simulink model "AC_SYS_SS"  (R2023b)
settings: Solver=FixedStepDiscrete  StartTime=0.0  StopTime=2  FixedStep=Ts_Power  RelTol=1e-4  EnableMultiTasking=on
PreLoadFcn:
  | HVDCMMCInterconnectionParam
StartFcn:
  | tic
StopFcn:
  | toc
values from neighbouring files (symbols this model uses):
  C_PM = 1.758e-3    (= 0.001758)    [HVDCMMCInterconnectionParam.m]
  D_R = 0.001    [HVDCMMCInterconnectionParam.m]
  D_Rs = 1e8    (= 100000000)    [HVDCMMCInterconnectionParam.m]
  Fnom = 50    [HVDCMMCInterconnectionParam.m]
  HRM = 2    [HVDCMMCInterconnectionParam.m]
  Limits_Qreg = [ 0.25, -0.25 ]    [HVDCMMCInterconnectionParam.m]
  Nb_PM = 36    [HVDCMMCInterconnectionParam.m]
  P_Ld1 = Psc/30    (= 666666666.667)    [HVDCMMCInterconnectionParam.m]
  Slope_Pref = 0.5    [HVDCMMCInterconnectionParam.m]
  Slope_Qref = 0.5    [HVDCMMCInterconnectionParam.m]
  Slope_Vdc_ref = Vnom_dc/5    (= 128000)    [HVDCMMCInterconnectionParam.m]
  Tbrk1_On = 0.1    [HVDCMMCInterconnectionParam.m]
  Tbrk2_On = 1.0    (= 1)    [HVDCMMCInterconnectionParam.m]
  Tdeblock = 1.5    [HVDCMMCInterconnectionParam.m]
  Tfault = 9999    [HVDCMMCInterconnectionParam.m]
  Ton_Converter2 = 4    [HVDCMMCInterconnectionParam.m]
  Ton_PQreg = 4    [HVDCMMCInterconnectionParam.m]
  Ton_VDCreg = 1.5    [HVDCMMCInterconnectionParam.m]
  Ts = Ts_Control    (= 4e-05)    [HVDCMMCInterconnectionParam.m]
  Ts_Power = 20e-6    (= 2e-05)    [HVDCMMCInterconnectionParam.m]
  Vb_dc = Vnom_dc    (= 640000)    [HVDCMMCInterconnectionParam.m]
  Vnom_dc = 640e3    (= 640000)    [HVDCMMCInterconnectionParam.m]
  Vnom_prim = 400e3    (= 400000)    [HVDCMMCInterconnectionParam.m]
  Vnom_sec = 333e3    (= 333000)    [HVDCMMCInterconnectionParam.m]
  w = 2*pi*Fnom    (= 314.159265359)    [HVDCMMCInterconnectionParam.m]
undefined symbols (not defined in the file or in its folder): ACSYS_T, DiscIntNeverNeededParam, Discrete, Pcc, sps_AC, spsDiodeModel
libraries: simulink x12, spsThreePhaseSeriesRLCBranchLib x7, spsGroundLib x3, spsControlledVoltageSourceLib x3, spsMultimeterLib x2, spsThreePhaseVIMeasurementLib x2, spsThreePhaseBreakerLib x1, spsThreePhaseSeriesRLCLoadLib x1, spspowerguiLib x1
(part 2 of 2)

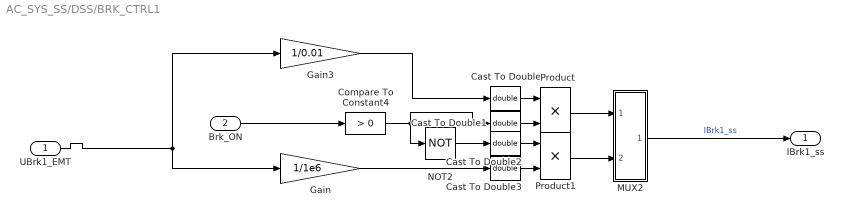
== system AC_SYS_SS/DSS/BRK_CTRL1 ==
  UBrk1_EMT : Inport
  Brk_ON : Inport  Port=2
  Cast To Double{,1..3} (4 alike) : DataTypeConversion  OutDataTypeStr=double  SaturateOnIntegerOverflow=off  RndMeth=Floor
  Compare To Constant4 : simulink/Logic and Bit Operations/Compare To Constant  relop=>  const=0  OutDataTypeStr=boolean
  Gain : Gain  Gain=1/1e6
  Gain3 : Gain  Gain=1/0.01
  MUX2 : Subsystem
  NOT2 : Logic  Operator=NOT  IconShape=distinctive  AllPortsSameDT=off  OutDataTypeStr=boolean
  Product : Product
  Product1 : Product
  IBrk1_ss : Outport
  wires:
  Cast To Double1/1 -> Product/2
  Product1/1 -> MUX2/2(In2)
  UBrk1_EMT/1 -> Gain3/1, Gain/1
  Compare To Constant4/1 -> Cast To Double1/1, NOT2/1
  Product/1 -> MUX2/1(In1)
  Gain/1 -> Cast To Double3/1
  NOT2/1 -> Cast To Double2/1
  Cast To Double/1 -> Product/1
  Gain3/1 -> Cast To Double/1
  Cast To Double3/1 -> Product1/2
  Brk_ON/1 -> Compare To Constant4/1
  Cast To Double2/1 -> Product1/1
  MUX2/1(Out1) -> IBrk1_ss/1  "IBrk1_ss"

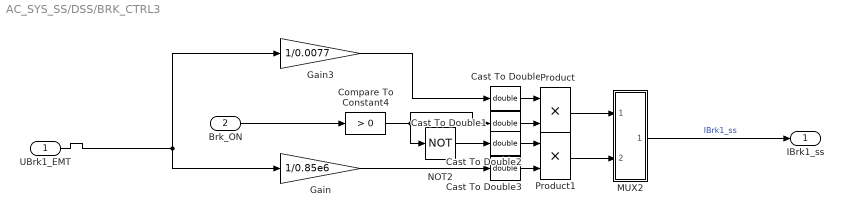
== system AC_SYS_SS/DSS/BRK_CTRL3 ==
  UBrk1_EMT : Inport
  Brk_ON : Inport  Port=2
  Cast To Double{,1..3} (4 alike) : DataTypeConversion  OutDataTypeStr=double  SaturateOnIntegerOverflow=off  RndMeth=Floor
  Compare To Constant4 : simulink/Logic and Bit Operations/Compare To Constant  relop=>  const=0  OutDataTypeStr=boolean
  Gain : Gain  Gain=1/0.85e6
  Gain3 : Gain  Gain=1/0.0077
  MUX2 : Subsystem
  NOT2 : Logic  Operator=NOT  IconShape=distinctive  AllPortsSameDT=off  OutDataTypeStr=boolean
  Product : Product
  Product1 : Product
  IBrk1_ss : Outport
  wires:
  Cast To Double1/1 -> Product/2
  Product1/1 -> MUX2/2(In2)
  UBrk1_EMT/1 -> Gain3/1, Gain/1
  Compare To Constant4/1 -> Cast To Double1/1, NOT2/1
  Product/1 -> MUX2/1(In1)
  Gain/1 -> Cast To Double3/1
  NOT2/1 -> Cast To Double2/1
  Cast To Double/1 -> Product/1
  Gain3/1 -> Cast To Double/1
  Cast To Double3/1 -> Product1/2
  Brk_ON/1 -> Compare To Constant4/1
  Cast To Double2/1 -> Product1/1
  MUX2/1(Out1) -> IBrk1_ss/1  "IBrk1_ss"

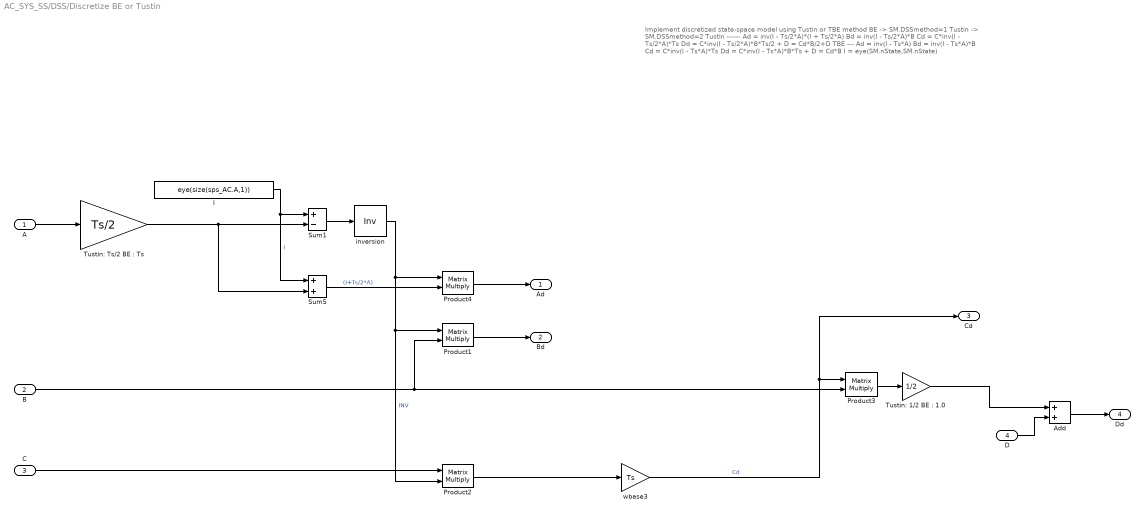
== system AC_SYS_SS/DSS/Discretize BE or Tustin ==
  note: Implement discretized state-space model using Tustin or TBE method
      |
      | BE      -> SM.DSSmethod=1
      | Tustin  -> SM.DSSmethod=2
      |
      |
      | Tustin
      | ------
      | Ad = inv(I - Ts/2*A)*(I + Ts/2*A)
      | Bd = inv(I - Ts/2*A)*B
      | Cd = C*inv(I - Ts/2*A)*Ts
      | Dd = C*inv(I - Ts/2*A)*B*Ts/2  + D  =  Cd*B/2+D
      |
      | TBE
      | ---
      | Ad = inv(I - Ts*A)
      | Bd = inv(I - Ts*A)*B
      | Cd = C*inv(I - Ts*A)*Ts
      | Dd = C*inv(I - Ts*A)*B*Ts  + D  =  Cd*B
      |
      | I = eye(SM.nState,SM.nState)
  A : Inport
  B : Inport  Port=2
  C : Inport  Port=3
  D : Inport  Port=4
  Add : Sum
  I : Constant  Value=eye(size(sps_AC.A,1))
  Product{1..4} (4 alike) : Product  Multiplication=Matrix(*)  SaturateOnIntegerOverflow=on  OutDataTypeStr=Inherit: Same as first input
  Sum1 : Sum  Inputs=+-  SaturateOnIntegerOverflow=on
  Sum5 : Sum  SaturateOnIntegerOverflow=on
  "Tustin: 1/2 BE : 1.0" : Gain  Gain=1/2  SaturateOnIntegerOverflow=on  OutDataTypeStr=Inherit: Same as input  ParamDataTypeStr=Inherit: Same as input
  "Tustin: Ts/2 BE : Ts" : Gain  Gain=Ts/2  SaturateOnIntegerOverflow=on  OutDataTypeStr=Inherit: Same as input  ParamDataTypeStr=Inherit: Same as input
  inversion : Product  Inputs=/  Multiplication=Matrix(*)  RndMeth=Zero
  wbase3 : Gain  Gain=Ts  SaturateOnIntegerOverflow=on  OutDataTypeStr=Inherit: Same as input  ParamDataTypeStr=Inherit: Same as input
  Ad : Outport  VectorParamsAs1DForOutWhenUnconnected=off
  Bd : Outport  Port=2  VectorParamsAs1DForOutWhenUnconnected=off
  Cd : Outport  Port=3  VectorParamsAs1DForOutWhenUnconnected=off
  Dd : Outport  Port=4  VectorParamsAs1DForOutWhenUnconnected=off
  wires:
  wbase3/1 -> Product3/1, Cd/1  "Cd"
  Product2/1 -> wbase3/1
  "Tustin: 1/2 BE : 1.0"/1 -> Add/1
  Product3/1 -> "Tustin: 1/2 BE : 1.0"/1
  C/1 -> Product2/1
  B/1 -> Product3/2, Product1/2
  Product1/1 -> Bd/1
  Sum5/1 -> Product4/2  "(I+Ts/2*A)"
  inversion/1 -> Product4/1, Product1/1, Product2/2  "INV"
  Sum1/1 -> inversion/1
  I/1 -> Sum1/1, Sum5/1  "I"
  A/1 -> "Tustin: Ts/2 BE : Ts"/1
  Product4/1 -> Ad/1
  "Tustin: Ts/2 BE : Ts"/1 -> Sum5/2, Sum1/2
  Add/1 -> Dd/1
  D/1 -> Add/2

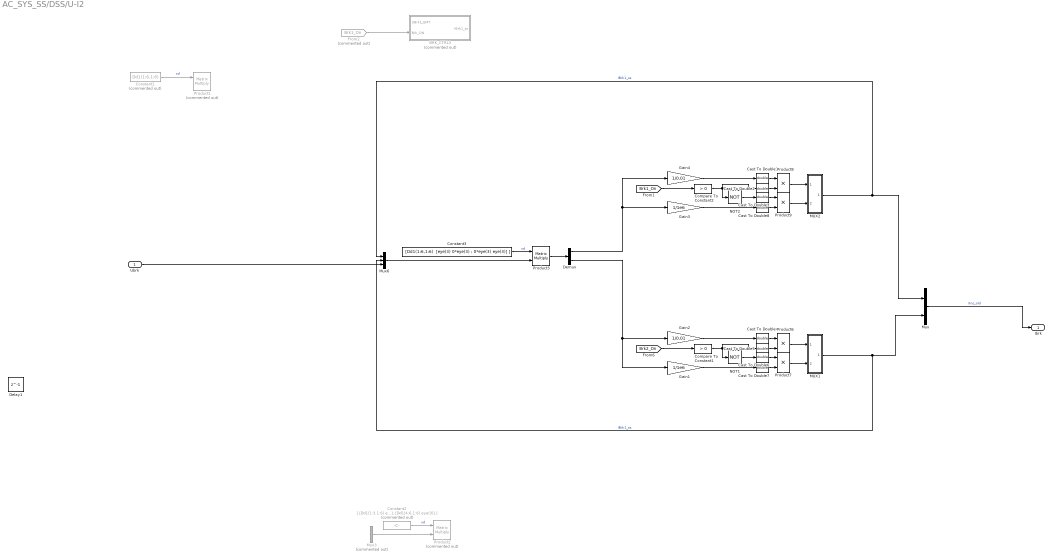
== system AC_SYS_SS/DSS/U-I2 ==
  Ubrk : Inport
  BRK_CTRL3 : Subsystem  Commented=on
  Cast To Double{1..8} (8 alike) : DataTypeConversion  OutDataTypeStr=double  SaturateOnIntegerOverflow=off  RndMeth=Floor
  Compare To Constant1 : simulink/Logic and Bit Operations/Compare To Constant  relop=>  const=0  OutDataTypeStr=boolean
  Compare To Constant2 : simulink/Logic and Bit Operations/Compare To Constant  relop=>  const=0  OutDataTypeStr=boolean
  Constant1 : Constant  Commented=on  Value=Dd1(1:6,1:6)
  Constant2 : Constant  Commented=on  Value=[ [Dd1(1:3,1:6) eye(3)]; [Dd1(4:6,1:6) eye(3)] ]
  Constant3 : Constant  Value="[Dd1(1:6,1:6)  [eye(3) 0*eye(3) ; 0*eye(3) eye(3)] ]"
  Delay1 : Delay  DelayLength=1  SampleTime=Ts_Power
  Demux : Demux  Outputs=2
  From2 : From  Commented=on  GotoTag=Brk1_On  TagVisibility=global
  Gain1 : Gain  Gain=1/1e6
  Gain2 : Gain  Gain=1/0.01
  Gain3 : Gain  Gain=1/1e6
  Gain4 : Gain  Gain=1/0.01
  MUX1 : Subsystem
  MUX2 : Subsystem
  Mux : Mux  Inputs=2
  Mux3 : Mux  Commented=on  Inputs=2
  Mux6 : Mux  Inputs=3
  NOT1 : Logic  Operator=NOT  IconShape=distinctive  AllPortsSameDT=off  OutDataTypeStr=boolean
  NOT2 : Logic  Operator=NOT  IconShape=distinctive  AllPortsSameDT=off  OutDataTypeStr=boolean
  Product1 : Product  Commented=on  Multiplication=Matrix(*)  SaturateOnIntegerOverflow=on  OutDataTypeStr=Inherit: Same as first input
  Product2 : Product  Commented=on  Multiplication=Matrix(*)  SaturateOnIntegerOverflow=on  OutDataTypeStr=Inherit: Same as first input
  Product3 : Product  Multiplication=Matrix(*)  SaturateOnIntegerOverflow=on  OutDataTypeStr=Inherit: Same as first input
  Product{6..9} (4 alike) : Product
  Ibrk : Outport
  wires:
  Mux/1 -> Ibrk/1  "Xns_old"
  Constant1/1 -> Product1/1  "xd"
  Cast To Double7/1 -> Product7/2
  Cast To Double6/1 -> Product7/1
  Gain2/1 -> Cast To Double4/1
  Compare To Constant1/1 -> Cast To Double5/1, NOT1/1
  NOT1/1 -> Cast To Double6/1
  Gain1/1 -> Cast To Double7/1
  Cast To Double5/1 -> Product6/2
  Cast To Double4/1 -> Product6/1
  [Brk2_On] -> Compare To Constant1/1
  Demux/2 -> Gain1/1, Gain2/1
  MUX1/1(UBrk1_EMT) -> Mux6/2, Mux/2  "IBrk1_ss"
  Product6/1 -> MUX1/1(In1)
  Product7/1 -> MUX1/2(In2)
  From2/1 -> BRK_CTRL3/2(Brk_ON)
  Cast To Double1/1 -> Product8/1
  Cast To Double2/1 -> Product8/2
  Gain3/1 -> Cast To Double8/1
  NOT2/1 -> Cast To Double3/1
  Cast To Double8/1 -> Product9/2
  Cast To Double3/1 -> Product9/1
  [Brk1_On] -> Compare To Constant2/1
  MUX2/1(UBrk1_EMT) -> Mux6/1, Mux/1  "IBrk1_ss"
  Gain4/1 -> Cast To Double1/1
  Product8/1 -> MUX2/1(In1)
  Compare To Constant2/1 -> Cast To Double2/1, NOT2/1
  Product9/1 -> MUX2/2(In2)
  ? -> Mux3/1
  ? -> Mux3/2
  Mux3/1 -> Product2/2
  Constant2/1 -> Product2/1  "xd"
  Mux6/1 -> Product3/2
  Constant3/1 -> Product3/1  "xd"
  Product3/1 -> Demux/1
  Demux/1 -> Gain4/1, Gain3/1
  Ubrk/1 -> Mux6/3

== system AC_SYS_SS/DSS/BRK_CTRL1/MUX2 ==
  In1 : Inport
  In2 : Inport  Port=2
  Demux4 : Demux  Outputs=3
  Demux5 : Demux  Outputs=3
  Mux13 : Mux  Inputs=2
  Mux14 : Mux  Inputs=2
  Mux15 : Mux  Inputs=3
  Mux8 : Mux  Inputs=2
  Sum1 : Sum  Inputs=1  InputSameDT=on  SaturateOnIntegerOverflow=on  OutDataTypeStr=Inherit: Same as first input
  Sum4 : Sum  Inputs=1  InputSameDT=on  SaturateOnIntegerOverflow=on  OutDataTypeStr=Inherit: Same as first input
  Sum5 : Sum  Inputs=1  InputSameDT=on  SaturateOnIntegerOverflow=on  OutDataTypeStr=Inherit: Same as first input
  Out1 : Outport
  wires:
  Demux5/3 -> Mux14/2
  In1/1 -> Demux4/1
  Demux4/1 -> Mux8/1
  Demux5/1 -> Mux8/2
  In2/1 -> Demux5/1
  Sum1/1 -> Mux15/1
  Demux5/2 -> Mux13/2
  Mux14/1 -> Sum5/1
  Mux8/1 -> Sum1/1
  Demux4/2 -> Mux13/1
  Mux13/1 -> Sum4/1
  Sum5/1 -> Mux15/3
  Sum4/1 -> Mux15/2
  Demux4/3 -> Mux14/1
  Mux15/1 -> Out1/1

== system AC_SYS_SS/DSS/BRK_CTRL3/MUX2 ==
  In1 : Inport
  In2 : Inport  Port=2
  Demux4 : Demux  Outputs=3
  Demux5 : Demux  Outputs=3
  Mux13 : Mux  Inputs=2
  Mux14 : Mux  Inputs=2
  Mux15 : Mux  Inputs=3
  Mux8 : Mux  Inputs=2
  Sum1 : Sum  Inputs=1  InputSameDT=on  SaturateOnIntegerOverflow=on  OutDataTypeStr=Inherit: Same as first input
  Sum4 : Sum  Inputs=1  InputSameDT=on  SaturateOnIntegerOverflow=on  OutDataTypeStr=Inherit: Same as first input
  Sum5 : Sum  Inputs=1  InputSameDT=on  SaturateOnIntegerOverflow=on  OutDataTypeStr=Inherit: Same as first input
  Out1 : Outport
  wires:
  Demux5/3 -> Mux14/2
  In1/1 -> Demux4/1
  Demux4/1 -> Mux8/1
  Demux5/1 -> Mux8/2
  In2/1 -> Demux5/1
  Sum1/1 -> Mux15/1
  Demux5/2 -> Mux13/2
  Mux14/1 -> Sum5/1
  Mux8/1 -> Sum1/1
  Demux4/2 -> Mux13/1
  Mux13/1 -> Sum4/1
  Sum5/1 -> Mux15/3
  Sum4/1 -> Mux15/2
  Demux4/3 -> Mux14/1
  Mux15/1 -> Out1/1

== system AC_SYS_SS/DSS/U-I2/BRK_CTRL3 ==
  UBrk1_EMT : Inport
  Brk_ON : Inport  Port=2
  Cast To Double{,1..3} (4 alike) : DataTypeConversion  OutDataTypeStr=double  SaturateOnIntegerOverflow=off  RndMeth=Floor
  Compare To Constant4 : simulink/Logic and Bit Operations/Compare To Constant  relop=>  const=0  OutDataTypeStr=boolean
  Gain : Gain  Gain=1/1e6
  Gain3 : Gain  Gain=1/0.01
  MUX2 : Subsystem
  NOT2 : Logic  Operator=NOT  IconShape=distinctive  AllPortsSameDT=off  OutDataTypeStr=boolean
  Product : Product
  Product1 : Product
  IBrk1_ss : Outport
  wires:
  Cast To Double1/1 -> Product/2
  Product1/1 -> MUX2/2(In2)
  UBrk1_EMT/1 -> Gain3/1, Gain/1
  Compare To Constant4/1 -> Cast To Double1/1, NOT2/1
  Product/1 -> MUX2/1(In1)
  Gain/1 -> Cast To Double3/1
  NOT2/1 -> Cast To Double2/1
  Cast To Double/1 -> Product/1
  Gain3/1 -> Cast To Double/1
  Cast To Double3/1 -> Product1/2
  Brk_ON/1 -> Compare To Constant4/1
  Cast To Double2/1 -> Product1/1
  MUX2/1(Out1) -> IBrk1_ss/1  "IBrk1_ss"

== system AC_SYS_SS/DSS/U-I2/MUX1 ==
  In1 : Inport
  In2 : Inport  Port=2
  Demux4 : Demux  Outputs=3
  Demux5 : Demux  Outputs=3
  Mux13 : Mux  Inputs=2
  Mux14 : Mux  Inputs=2
  Mux15 : Mux  Inputs=3
  Mux8 : Mux  Inputs=2
  Sum1 : Sum  Inputs=1  InputSameDT=on  SaturateOnIntegerOverflow=on  OutDataTypeStr=Inherit: Same as first input
  Sum4 : Sum  Inputs=1  InputSameDT=on  SaturateOnIntegerOverflow=on  OutDataTypeStr=Inherit: Same as first input
  Sum5 : Sum  Inputs=1  InputSameDT=on  SaturateOnIntegerOverflow=on  OutDataTypeStr=Inherit: Same as first input
  UBrk1_EMT : Outport
  wires:
  Demux5/3 -> Mux14/2
  In1/1 -> Demux4/1
  Demux4/1 -> Mux8/1
  Demux5/1 -> Mux8/2
  In2/1 -> Demux5/1
  Sum1/1 -> Mux15/1
  Demux5/2 -> Mux13/2
  Mux14/1 -> Sum5/1
  Mux8/1 -> Sum1/1
  Demux4/2 -> Mux13/1
  Mux13/1 -> Sum4/1
  Sum5/1 -> Mux15/3
  Sum4/1 -> Mux15/2
  Demux4/3 -> Mux14/1
  Mux15/1 -> UBrk1_EMT/1

== system AC_SYS_SS/DSS/U-I2/MUX2 ==
  In1 : Inport
  In2 : Inport  Port=2
  Demux4 : Demux  Outputs=3
  Demux5 : Demux  Outputs=3
  Mux13 : Mux  Inputs=2
  Mux14 : Mux  Inputs=2
  Mux15 : Mux  Inputs=3
  Mux8 : Mux  Inputs=2
  Sum1 : Sum  Inputs=1  InputSameDT=on  SaturateOnIntegerOverflow=on  OutDataTypeStr=Inherit: Same as first input
  Sum4 : Sum  Inputs=1  InputSameDT=on  SaturateOnIntegerOverflow=on  OutDataTypeStr=Inherit: Same as first input
  Sum5 : Sum  Inputs=1  InputSameDT=on  SaturateOnIntegerOverflow=on  OutDataTypeStr=Inherit: Same as first input
  UBrk1_EMT : Outport
  wires:
  Demux5/3 -> Mux14/2
  In1/1 -> Demux4/1
  Demux4/1 -> Mux8/1
  Demux5/1 -> Mux8/2
  In2/1 -> Demux5/1
  Sum1/1 -> Mux15/1
  Demux5/2 -> Mux13/2
  Mux14/1 -> Sum5/1
  Mux8/1 -> Sum1/1
  Demux4/2 -> Mux13/1
  Mux13/1 -> Sum4/1
  Sum5/1 -> Mux15/3
  Sum4/1 -> Mux15/2
  Demux4/3 -> Mux14/1
  Mux15/1 -> UBrk1_EMT/1

== system AC_SYS_SS/DSS/U-I2/BRK_CTRL3/MUX2 ==
  In1 : Inport
  In2 : Inport  Port=2
  Demux4 : Demux  Outputs=3
  Demux5 : Demux  Outputs=3
  Mux13 : Mux  Inputs=2
  Mux14 : Mux  Inputs=2
  Mux15 : Mux  Inputs=3
  Mux8 : Mux  Inputs=2
  Sum1 : Sum  Inputs=1  InputSameDT=on  SaturateOnIntegerOverflow=on  OutDataTypeStr=Inherit: Same as first input
  Sum4 : Sum  Inputs=1  InputSameDT=on  SaturateOnIntegerOverflow=on  OutDataTypeStr=Inherit: Same as first input
  Sum5 : Sum  Inputs=1  InputSameDT=on  SaturateOnIntegerOverflow=on  OutDataTypeStr=Inherit: Same as first input
  Out1 : Outport
  wires:
  Demux5/3 -> Mux14/2
  In1/1 -> Demux4/1
  Demux4/1 -> Mux8/1
  Demux5/1 -> Mux8/2
  In2/1 -> Demux5/1
  Sum1/1 -> Mux15/1
  Demux5/2 -> Mux13/2
  Mux14/1 -> Sum5/1
  Mux8/1 -> Sum1/1
  Demux4/2 -> Mux13/1
  Mux13/1 -> Sum4/1
  Sum5/1 -> Mux15/3
  Sum4/1 -> Mux15/2
  Demux4/3 -> Mux14/1
  Mux15/1 -> Out1/1

== matlab function AC_SYS_SS/MATLAB Function ==
  data: usw output; Id input; status output; Vd input
function [usw, status]   = DFcn(Id, Vd)

    persistent SW;
    
    if(isempty(SW)) SW = 1; end
    
    
    if(Id<=0 && SW == 1)
    
        SW = 0;
    elseif( (Id>0 && SW == 0) || (Vd > 0.7 && SW == 0 && Id>eps) )
        SW = 1;
    end
    
    status = SW;
    usw = Vd;

end

== matlab function AC_SYS_SS/MATLAB Function2 ==
  data: Usm input; Uref input; UDt output; Stt output; Ip input; Ic input; UDb output; Stb output; IDt output; IDb output; Vbl output; Ts parameter; D_R parameter; D_Rs parameter; Nb_SM parameter; C parameter; Vin output
function [UDt, Stt, UDb, Stb, IDt, IDb, Vbl, Vin]   = DFcn(Usm, Uref, Ip, Ic, Ts, D_R, D_Rs, Nb_SM, C)

    UDt = 0; UDb = 0; Stt = 0; Stb = 0;

    Ib    = 0;
    Vbl = 0;
    Vin = 0;
    IDt = 0;
    IDb = 0;
    
    persistent timer;
    persistent Usm_old;
    persistent Ip_old;
    persistent Ic_old;
    persistent SWt;
    persistent SWb;

    persistent Uc_old;
    persistent Uc;
    persistent x_old;
    persistent Req;
    
    if(isempty(timer)) 
        timer = 0; 
        Usm_old = 0;
        Ip_old = 0;
        Ic_old = 0;
        SWt = 0;
        SWb = 0;
        Uc_old = 0;
        Uc = 0;
        x_old = 0;
        Req = D_R*D_Rs/(D_R+D_Rs);
    end
    
    timer = timer + Ts;

%%%%%%%%%%%%%%% Calc Vin & Vbl %%%%%%%%%%%%%%%
    %x = Nb_SM*(Ip_old*Uref(1)+Ic_old*Uref(2))/(C*Nb_SM);
    x = Nb_SM*(Ip*Uref(1)+Ic*Uref(2))/(C*Nb_SM);

    Uc = (Ts/2)*(x+x_old) + Uc_old;
    
    Vin = Uc*Uref(1)*Nb_SM;
    Vbl = Uc*Uref(2)*Nb_SM;


    x_old = x;
    Uc_old = Uc;
%%%%%%%%%%%%%%%%%%%%%%%%%%%%%%


    Ib = Ip-D_Rs/(D_R+D_Rs)*Ic;


    if(Uref(2) > 0)

        if(Ic < 0)
            UDt = Usm - Vbl;
        else
            UDt = Ic*Req;
        end
    
        if(Ib > 0)
            UDb = -Usm;
        else
            UDb = -Ib*Req;
        end

        1==1;
    
        if(-0.0001 + D_Rs/(D_R+D_Rs)*Ic_old <= 0 && SWt == 1)
            SWt = 0;
        elseif(-0.0001 + D_Rs/(D_R+D_Rs)*Ic > 0 && SWt == 0) 
            SWt = 1;
        end
    
        if(Ib<=0 && SWb == 0 && SWt == 0)
            SWb = 1;
        elseif( (Ib > -eps && SWb == 1 && Vbl > 0 && Ip < 0))
            SWb = 0;
        end

    else
        UDt =  Ip*(D_Rs/2)*D_R/(D_Rs/2+D_R);
        UDb = -UDt;


        if((0.1+Ib<=0 || Ip<0) && SWb == 0)
            SWb = 1;
            SWt = 0;
        elseif( (Ip>0 || -0.1 + Ic >= 0) && SWb == 1)
            SWb = 0;
            SWt = 1;
        end


    end




    IDt = SWt * UDt / D_R;
    if(IDt<0) IDt = 0; end

    IDb = SWb * UDb / D_R;
    if(IDb<0) IDb = 0; end


    Usm_old = Usm;
    Ip_old = Ip;
    Ic_old = Ic;



    Stt =  SWt;
    Stb = SWb;

end


    % if(SWt>0.5)
    %     IDt = UDt / D_R;
    %     if(IDt<0) IDt = 0; end
    % else
    %     IDt = 0;
    % end
    % 
    % if(SWb>0.5)
    %     IDb = UDb / D_R;
    %     if(IDb<0) IDb = 0; end
    % else
    %     IDb = 0;
    % end


    % persistent SW;
    % 
    % if(isempty(SW)) SW = 1; end
    % 
    % 
    % if(Id<=0 && SW == 1)
    % 
    %     SW = 0;
    % elseif( (Id>0 && SW == 0) || (Vd > 0 && SW == 0 && Id>eps) )
    %     SW = 1;
    % end
    % 
    % status = SW;
    % usw = Vd;

== matlab function AC_SYS_SS/DQn->ABC ==
  settings: updateMethod=DISCRETE
  data: Xdcpnz_c input; tho input; Xabc output; N parameter
%function abc = Mult(Z0,Zdp,Zqp,Zdn,Zqn,Zdz,Zqz,th, N)
function Xabc = dqn2abc(Xdcpnz_c,tho,N)

    persistent Sas;
    persistent Ssa;

    if(isempty(Sas)) 
        a = -0.5+0.866i;
        a2 = -0.5-0.866i;
        Sas = [1,a,a2;1,a2,a;1,1,1]/3;
        Ssa = eye(3)/(Sas);
    end

    Xabc = zeros(3,1);

    for i = 1 : N+1
    
    
        if(i>1)
            h = i-1;
    
            th = h*tho;
        
            mag_p = abs(Xdcpnz_c(1,i));
            ang_p = angle(Xdcpnz_c(1,i));
            mag_n = abs(Xdcpnz_c(2,i));
            ang_n = angle(Xdcpnz_c(2,i));
            mag_z = abs(Xdcpnz_c(3,i));
            ang_z = angle(Xdcpnz_c(3,i));
            
            abc3p = mag_p*[sin(th+ang_p) ; sin(th+ang_p-2*pi/3) ; sin(th+ang_p+2*pi/3) ];
            abc3n = mag_n*[sin(th+ang_n) ; sin(th+ang_n+2*pi/3) ; sin(th+ang_n-2*pi/3) ];
            abc3z = mag_z*[sin(th+ang_z) ; sin(th+ang_z)        ; sin(th+ang_z)  ];
        
            Xabc = Xabc + abc3p+abc3n+abc3z;
        else
            Xabc = Xabc + real(Ssa*(Xdcpnz_c(:,1)));
        
        end
    
        
    end

end
